simulink model "ComTest"  (R2025a)
settings: Solver=VariableStepAuto  StartTime=0.0  StopTime=1  RelTol=1e-3
libraries: instrumentlib x4
settings Model: Creator=changhong  LastModifiedBy=changhong

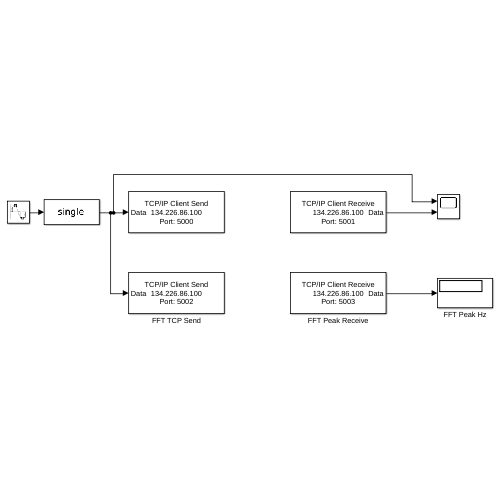
[thumbnail: Simulink's stored preview of the top-level diagram]
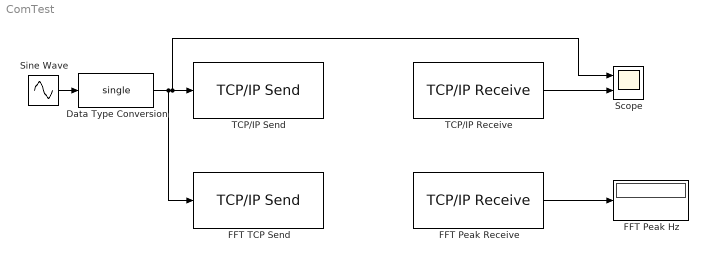
== system ComTest ==
  Data Type Conversion : DataTypeConversion  OutDataTypeStr=single  SaturateOnIntegerOverflow=off  RndMeth=Floor
  FFT Peak Hz : Display
  FFT Peak Receive : instrumentlib/TCP//IP Receive  Priority=20  Host=134.226.86.100  Port=5003  DataSize=[1, 1]  DataType=single  ASCIIFormatting=%f  Terminator=LF  CustomTerminator=10  ByteOrder=little-endian  EnableBlockingMode=on  Timeout=10  SampleTime=1/4000  SimulateUsing=Interpreted execution
  FFT TCP Send : instrumentlib/TCP//IP Send  Priority=-9  Host=134.226.86.100  Port=5002  ByteOrder=little-endian  EnableBlockingMode=on  Timeout=10  TransferDelay=off  SimulateUsing=Interpreted execution
  Scope : Scope  NumInputPorts=2
      settings: ActiveDisplayYMinimum=-1.8031417735137669  ActiveDisplayYMaximum=1.2698598054298436
  Sine Wave : Sin  Frequency=100*pi  SampleTime=1/4000
  TCP/IP Receive : instrumentlib/TCP//IP Receive  Priority=10  Host=134.226.86.100  Port=5001  DataSize=[1, 1]  DataType=single  ASCIIFormatting=%f  Terminator=LF  CustomTerminator=10  ByteOrder=little-endian  EnableBlockingMode=on  Timeout=10  SampleTime=1/4000  SimulateUsing=Interpreted execution
  TCP/IP Send : instrumentlib/TCP//IP Send  Priority=-10  Host=134.226.86.100  Port=5000  ByteOrder=little-endian  EnableBlockingMode=on  Timeout=10  TransferDelay=off  SimulateUsing=Interpreted execution
  wires:
  Sine Wave/1 -> Data Type Conversion/1
  Data Type Conversion/1 -> Scope/1, TCP/IP Send/1, FFT TCP Send/1
  TCP/IP Receive/1 -> Scope/2
  FFT Peak Receive/1 -> FFT Peak Hz/1
